simulink model "Lab4Modelsp4"  (R2013b)
settings: Solver=ode45  StartTime=0.0  StopTime=10.0  RelTol=1e-3
libraries: simulink x2
settings Model: Creator=SuperUser  LastModifiedBy=Эдик
settings DataIOCC: SignalLoggingSaveFormat=ModelDataLogs
settings DebuggingCC: UnderspecifiedInitializationDetection=Simplified  MultiTaskDSMMsg=warning  MultiTaskCondExecSysMsg=none
settings RTWCC: IncludeERTFirstTime=on
settings GRTTargetCC: CodeReplacementLibrary=None  CPPClassGenCompliant=on

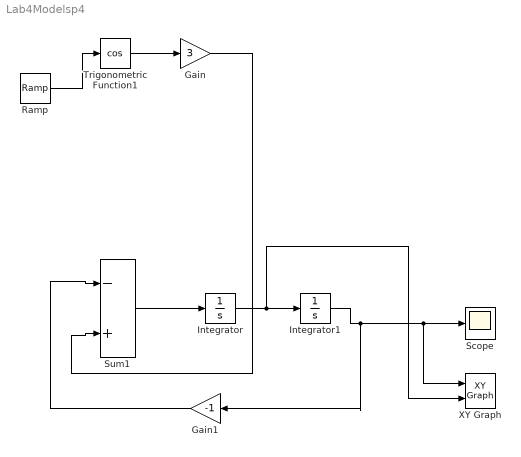
== system Lab4Modelsp4 ==
  Gain : Gain  Gain=3
  Gain1 : Gain  Gain=-1
  Integrator : Integrator  InitialCondition=4
  Integrator1 : Integrator  InitialCondition=1
  Ramp : simulink/Sources/Ramp  slope=1  start=0  X0=0
  Scope : Scope
  Sum1 : Sum  Inputs=-+
  Trigonometric Function1 : Trigonometry  Operator=cos
  XY Graph : simulink/Sinks/XY Graph  xmin=0  xmax=10  ymin=1  ymax=10  st=-1
  wires:
  Ramp/1 -> Trigonometric Function1/1
  Trigonometric Function1/1 -> Gain/1
  Gain/1 -> Sum1/2
  Sum1/1 -> Integrator/1
  Integrator1/1 -> Gain1/1, XY Graph/1, Scope/1
  Integrator/1 -> XY Graph/2, Integrator1/1
  Gain1/1 -> Sum1/1
